simulink model "SecureRoom_SubsystemTrigger"  (R2016a)
settings: Solver=FixedStepDiscrete  StartTime=0.0  StopTime=10.0  RelTol=1e-3
settings Model: Creator=Banna  LastModifiedBy=Banna
settings OptimizationCC: DefaultParameterBehavior=Inlined  InlineInvariantSignals=on  EnableMemcpy=off  OptimizeModelRefInitCode=on  LifeSpan=1
settings DebuggingCC: UnderspecifiedInitializationDetection=Classic  MergeDetectMultiDrivingBlocksExec=none
settings ModelReferenceCC: PropagateSignalLabelsOutOfModel=off
settings RTWCC: SystemTargetFile=ert.tlc  GenCodeOnly=on  TemplateMakefile=ert_default_tmf  GenerateReport=on  IncludeHyperlinkInReport=on  LaunchReport=on  GenerateTraceInfo=on  GenerateTraceReport=on  GenerateTraceReportSl=on  GenerateTraceReportSf=on  GenerateTraceReportEml=on
settings CodeAppCC: ForceParamTrailComments=on  IgnoreCustomStorageClasses=off  OperatorAnnotations=on  SimulinkDataObjDesc=on  SFDataObjDesc=on  MATLABFcnDesc=on  InsertBlockDesc=on  MATLABSourceComments=on
settings ERTTargetCC: GenerateSampleERTMain=on  InlinedParameterPlacement=NonHierarchical  ERTCustomFileTemplate=example_file_process.tlc

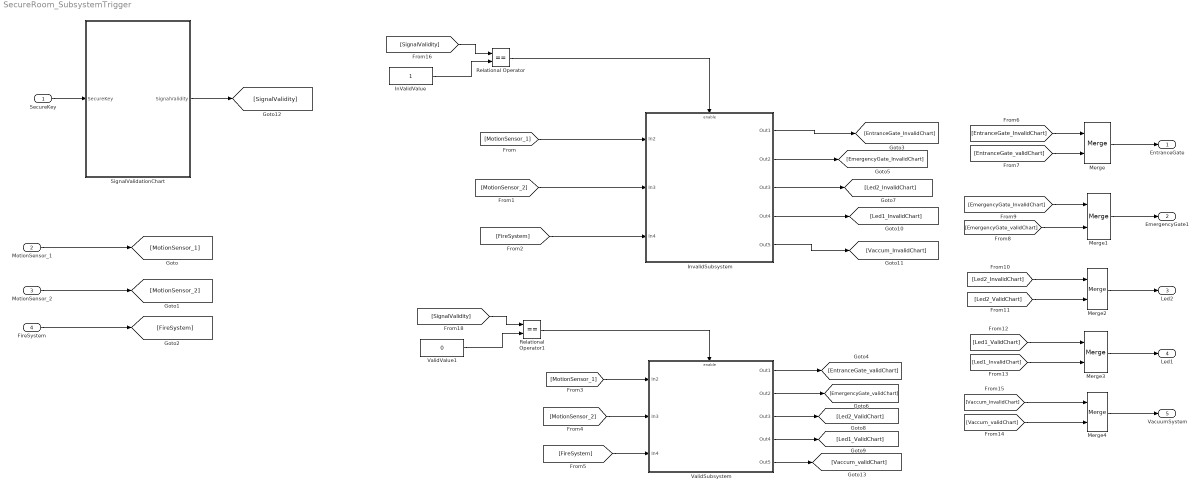
== system SecureRoom_SubsystemTrigger ==
  SecureKey : Inport
  MotionSensor_1 : Inport  Port=2
  MotionSensor_2 : Inport  Port=3
  FireSystem : Inport  Port=4
  InValidValue : Constant
  InvalidSubsystem : Subsystem
  Merge{,1..4} (5 alike) : Merge
  Relational Operator : RelationalOperator  Operator===  OutDataTypeStr=boolean
  Relational Operator1 : RelationalOperator  Operator===  OutDataTypeStr=boolean
  SignalValidationChart : Stateflow chart  TreatAsAtomicUnit=on
  ValidSubsystem : Subsystem
  ValidValue1 : Constant  Value=0
  EntranceGate : Outport
  EmergencyGate1 : Outport  Port=2
  Led2 : Outport  Port=3
  "Led1 " : Outport  Port=4
  VacuumSystem : Outport  Port=5
  wires:
  SecureKey/1 -> SignalValidationChart/1(SecureKey)
  MotionSensor_1/1 -> [MotionSensor_1]
  MotionSensor_2/1 -> [MotionSensor_2]
  FireSystem/1 -> [FireSystem]
  Merge/1 -> EntranceGate/1
  Merge1/1 -> EmergencyGate1/1
  Merge3/1 -> "Led1 "/1
  Merge2/1 -> Led2/1
  Merge4/1 -> VacuumSystem/1
  [EntranceGate_InvalidChart] -> Merge/1
  [EntranceGate_validChart] -> Merge/2
  [EmergencyGate_validChart] -> Merge1/2
  [EmergencyGate_InvalidChart] -> Merge1/1
  [Led2_InvalidChart] -> Merge2/1
  [Led2_ValidChart] -> Merge2/2
  [Led1_ValidChart] -> Merge3/1
  [Led1_InvalidChart] -> Merge3/2
  [Vaccum_validChart] -> Merge4/2
  [Vaccum_InvalidChart] -> Merge4/1
  [MotionSensor_1] -> InvalidSubsystem/1(In2)
  [MotionSensor_2] -> InvalidSubsystem/2(In3)
  [FireSystem] -> InvalidSubsystem/3(In4)
  InvalidSubsystem/1(Out1) -> [EntranceGate_InvalidChart]
  InvalidSubsystem/2(Out2) -> [EmergencyGate_InvalidChart]
  InvalidSubsystem/3(Out3) -> [Led2_InvalidChart]
  InvalidSubsystem/4(Out4) -> [Led1_InvalidChart]
  InvalidSubsystem/5(Out5) -> [Vaccum_InvalidChart]
  [MotionSensor_1] -> ValidSubsystem/1(In2)
  [MotionSensor_2] -> ValidSubsystem/2(In3)
  [FireSystem] -> ValidSubsystem/3(In4)
  ValidSubsystem/1(Out1) -> [EntranceGate_validChart]
  ValidSubsystem/2(Out2) -> [EmergencyGate_validChart]
  ValidSubsystem/3(Out3) -> [Led2_ValidChart]
  ValidSubsystem/4(Out4) -> [Led1_ValidChart]
  ValidSubsystem/5(Out5) -> [Vaccum_validChart]
  SignalValidationChart/1(SignalValidity) -> [SignalValidity]
  [SignalValidity] -> Relational Operator/1
  InValidValue/1 -> Relational Operator/2
  Relational Operator/1 -> InvalidSubsystem/Enable
  [SignalValidity] -> Relational Operator1/1
  ValidValue1/1 -> Relational Operator1/2
  Relational Operator1/1 -> ValidSubsystem/Enable

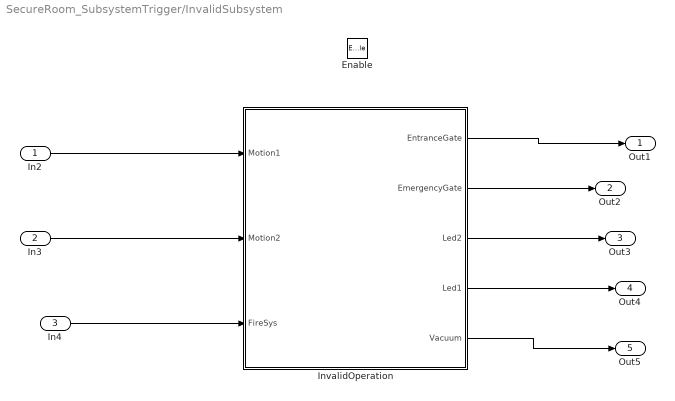
== system SecureRoom_SubsystemTrigger/InvalidSubsystem ==
  In2 : Inport
  In3 : Inport  Port=2
  In4 : Inport  Port=3
  Enable : EnablePort
  InvalidOperation : Stateflow chart  TreatAsAtomicUnit=on
  Out1 : Outport
  Out2 : Outport  Port=2
  Out3 : Outport  Port=3
  Out4 : Outport  Port=4
  Out5 : Outport  Port=5
  wires:
  In2/1 -> InvalidOperation/1(Motion1)
  In4/1 -> InvalidOperation/3(FireSys)
  In3/1 -> InvalidOperation/2(Motion2)
  InvalidOperation/1(EntranceGate) -> Out1/1
  InvalidOperation/5(Vacuum) -> Out5/1
  InvalidOperation/4(Led1) -> Out4/1
  InvalidOperation/2(EmergencyGate) -> Out2/1
  InvalidOperation/3(Led2) -> Out3/1

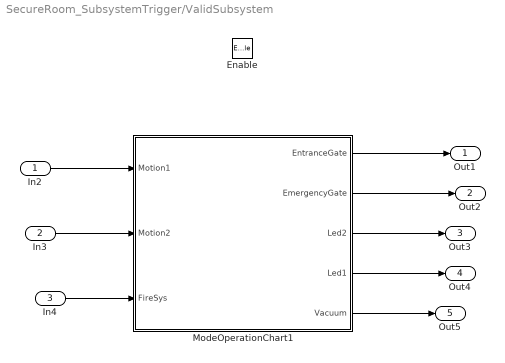
== system SecureRoom_SubsystemTrigger/ValidSubsystem ==
  In2 : Inport
  In3 : Inport  Port=2
  In4 : Inport  Port=3
  Enable : EnablePort
  ModeOperationChart1 : Stateflow chart  TreatAsAtomicUnit=on
  Out1 : Outport
  Out2 : Outport  Port=2
  Out3 : Outport  Port=3
  Out4 : Outport  Port=4
  Out5 : Outport  Port=5
  wires:
  ModeOperationChart1/1(EntranceGate) -> Out1/1
  ModeOperationChart1/5(Vacuum) -> Out5/1
  In2/1 -> ModeOperationChart1/1(Motion1)
  ModeOperationChart1/2(EmergencyGate) -> Out2/1
  ModeOperationChart1/3(Led2) -> Out3/1
  In3/1 -> ModeOperationChart1/2(Motion2)
  ModeOperationChart1/4(Led1) -> Out4/1
  In4/1 -> ModeOperationChart1/3(FireSys)

== stateflow chart SecureRoom_SubsystemTrigger/InvalidSubsystem/InvalidOperation ==
  state Invalid
    en:
    EntranceGate=0;
    EmergencyGate=0;
    Led1=0;
    Led2=0;
    Vacuum=0;
    du:
    ex:
  (default) -> Invalid
  data: EntranceGate output; EmergencyGate output; Motion1 input; Motion2 input; Led2 output; Led1 output; Vacuum output; EmergencyCounter local uint8; FireSys input

== stateflow chart SecureRoom_SubsystemTrigger/ValidSubsystem/ModeOperationChart1 ==
  state Room2
    en:
    Led1=0;
    Led2=1;
    Vacuum=0;
    EntranceGate=1;
    EmergencyGate=1;
    du:
    ex:
  state Room1
    en:
    Led1=1;
    Led2=0;
    Vacuum=0;
    EntranceGate=1;
    EmergencyGate=1;
    du:
    ex:
  state Emergency
    en:
    Led1=1;
    Led2=1;
    Vacuum=1;
    du:
    EmergencyCounter++;
    ex:
  state SystemLocked
    en:
    EntranceGate=0;
    EmergencyGate=0;
    du:
    ex:
  (default) -> Room1
  Room1 -> Room2 [order 1] : [Motion1==0 && Motion2==1]
  Room2 -> Room1 [order 1] : [Motion1==1 && Motion2==0]
  Room2 -> (junction 73) [order 2]
  Room1 -> (junction 74) [order 2]
  (junction 74) -> Emergency : [FireSys==1]
  (junction 73) -> Emergency : [FireSys==1]
  Emergency -> SystemLocked : [EmergencyCounter==5]
  data: EntranceGate output; EmergencyGate output; Motion1 input; Motion2 input; Led2 output; Led1 output; Vacuum output; EmergencyCounter local uint8; FireSys input

== stateflow chart SecureRoom_SubsystemTrigger/SignalValidationChart ==
  note: The added condition of "InvalidCounter<3"
      | to prevent counter increment if it reach value = 3
  (default) -> (junction 67) : /* Check on Key Validity */
  (junction 67) -> (junction 68) [order 1] : /*Check if key is invalid for times less than 3*/
      | [SecureKey==0 && InvalidCounter<3]
  (junction 67) -> (junction 69) [order 2]
  (junction 68) -> (junction 73) : /*Increment the error counter*/
      | {InvalidCounter++;}
  (junction 69) -> (junction 70) [order 1] : /*if the key is valid*/
      | [SecureKey==1 && InvalidCounter<3]
  (junction 69) -> (junction 71) [order 2] : /*Do nothing if the
      | Key is invalid for more than three times
      | , system is locked*/
  (junction 70) -> (junction 72) : /*reset the counter*/
      | {InvalidCounter=0;}
  (junction 72) -> (junction 71)
  (junction 73) -> (junction 72)
  (junction 71) -> (junction 45)
  (junction 45) -> (junction 46) [order 1] : /*Invalid Input for three times*/
      | [InvalidCounter==3]
  (junction 45) -> (junction 47) [order 2]
  (junction 46) -> (junction 54) : /*Report Invalid Signal to the System*/
      | {
      | SignalValidity=0;
      | }
  (junction 47) -> (junction 48) [order 1] : /*Invalid signal for time more than one*/
      | [InvalidCounter>0 && SecureKey==0]
  (junction 48) -> (junction 53) : /*Tempory Signal untill
      | signal became stable*/
      | /*do not trigger any event*/
  (junction 47) -> (junction 49) [order 2]
  (junction 49) -> (junction 50) [order 1] : /*Valid Input*/
      | [InvalidCounter==0]
  (junction 49) -> (junction 51) [order 2] : {/*Do Nothing*/;}
  (junction 50) -> (junction 52) : /*Report Valid Signal*/
      | {SignalValidity=1;}
  (junction 52) -> (junction 51)
  (junction 53) -> (junction 52)
  (junction 54) -> (junction 53)
  (junction 51) -> (junction 55)
  data: InvalidCounter local uint8; SecureKey input; SignalValidity output uint8
